simulink model "discrete_linear"  (R2017b)
settings: Solver=VariableStepAuto  StartTime=0.0  StopTime=70  RelTol=1e-3
values from neighbouring files (symbols this model uses):
  a1 = 0.44    [workspace.mat]    (also in workspace2.mat)
  a2 = 0.51    [workspace.mat]    (also in workspace2.mat)
  a3 = 0.48    [workspace.mat]    (also in workspace2.mat)
  a4 = -0.65    [workspace.mat]    (also in workspace2.mat)
  K = 2.5    [workspace.mat]    (also in workspace2.mat)
  T1 = 5    [workspace.mat]    (also in workspace2.mat)
  T2 = 10    [workspace.mat]    (also in workspace2.mat)
  Tp = 1    [workspace.mat]    (also in workspace2.mat)
  u_lin = 0.8    [workspace2.mat]
settings Model: Creator=gulin  LastModifiedBy=gulin

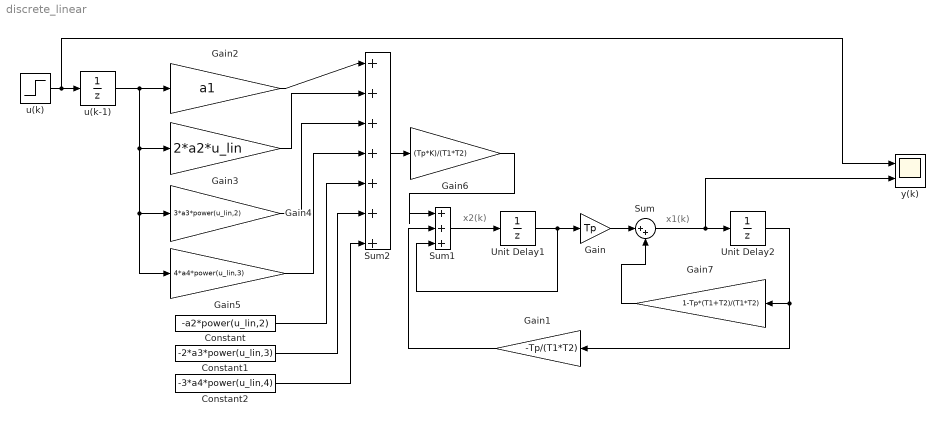
== system discrete_linear ==
  note: x1(k)
  note: x2(k)
  Constant : Constant  Value=-a2*power(u_lin,2)
  Constant1 : Constant  Value=-2*a3*power(u_lin,3)
  Constant2 : Constant  Value=-3*a4*power(u_lin,4)
  Gain : Gain  Gain=Tp
  Gain1 : Gain  Gain=-Tp/(T1*T2)
  Gain2 : Gain  Gain=a1
  Gain3 : Gain  Gain=2*a2*u_lin
  Gain4 : Gain  Gain=3*a3*power(u_lin,2)
  Gain5 : Gain  Gain=4*a4*power(u_lin,3)
  Gain6 : Gain  Gain=(Tp*K)/(T1*T2)
  Gain7 : Gain  Gain=1-Tp*(T1+T2)/(T1*T2)
  Sum : Sum  Inputs=|++
  Sum1 : Sum  Inputs=|+++
  Sum2 : Sum  Inputs=|+++++++
  Unit Delay1 : UnitDelay  SampleTime=Tp
  Unit Delay2 : UnitDelay  SampleTime=Tp
  u(k) : Step  After=-0.5  SampleTime=0
  u(k-1) : UnitDelay  SampleTime=Tp
  y(k) : Scope  NumInputPorts=2
  wires:
  Gain4/1 -> Sum2/3
  Gain3/1 -> Sum2/2
  Gain2/1 -> Sum2/1
  Gain5/1 -> Sum2/4
  Sum2/1 -> Gain6/1
  u(k-1)/1 -> Gain5/1, Gain4/1, Gain3/1, Gain2/1
  Sum1/1 -> Unit Delay1/1
  Unit Delay1/1 -> Gain/1, Sum1/3
  Gain/1 -> Sum/1
  Sum/1 -> y(k)/2, Unit Delay2/1
  Gain6/1 -> Sum1/1
  Unit Delay2/1 -> Gain1/1, Gain7/1
  Gain1/1 -> Sum1/2
  Gain7/1 -> Sum/2
  Constant/1 -> Sum2/5
  Constant1/1 -> Sum2/6
  Constant2/1 -> Sum2/7
  u(k)/1 -> y(k)/1, u(k-1)/1
